simulink model "TorqueControl"  (R2019a)
settings: Solver=FixedStepAuto  StartTime=0.0  StopTime=6  FixedStep=0.015  RelTol=1e-3
undefined symbols (not defined in the file): f_sw, Q_rr, r_c, r_D, u_ce0, u_D0
libraries: Lib_Solve_SSNRSolverJC_TMATS x2, simulink x1
settings Model: Creator=gfretti  LastModifiedBy=gfretti

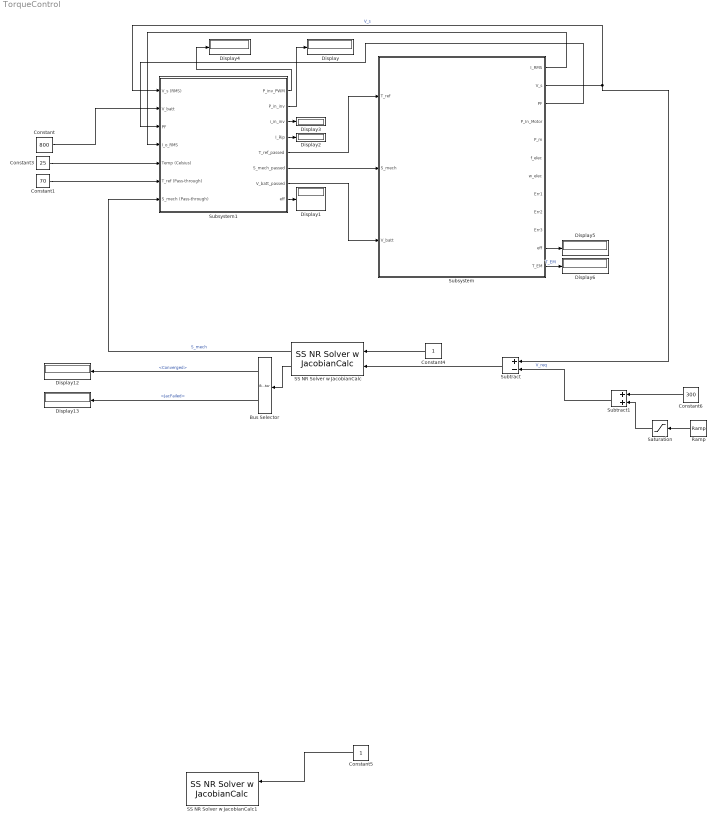
== system TorqueControl ==
  Bus Selector : BusSelector  OutputSignals=Converged,JacFailed
  Constant : Constant  Value=800
  Constant1 : Constant  Value=70
  Constant3 : Constant  Value=25
  Constant4 : Constant
  Constant5 : Constant
  Constant6 : Constant  Value=300
  Display{,1..6,12..13} (9 alike) : Display
  Ramp : simulink/Sources/Ramp  slope=25  start=2  InitialOutput=0
  SS NR Solver w JacobianCalc : Lib_Solve_SSNRSolverJC_TMATS/SS NR Solver w JacobianCalc  SJac_Per_M=[-0.1;-0.01;0.01;0.1]  SNR_IC_M=100  SNR_DX_M=100  SNR_Mx_M=100000  SNR_Mn_M=0.00001  SJacobianAttempts_M=2*10^5  Cond_Limits_M=0.01
  SS NR Solver w JacobianCalc1 : Lib_Solve_SSNRSolverJC_TMATS/SS NR Solver w JacobianCalc  SJac_Per_M=[-0.01;0.01]  SNR_IC_M=150  SNR_DX_M=100  SNR_Mx_M=100000  SNR_Mn_M=0.00001  SJacobianAttempts_M=20000  Cond_Limits_M=0.01
  Saturation : Saturate  UpperLimit=50
  Subsystem : Subsystem  mask{pp=2, flux_m=0.57773, R_s=0.032, L_s=0.00115, P_Fe_Nom=904.3614, S_nom=3000, T_nom=70, P_out_max=22000, I_max=36.5, P_in_max=30000, T_max=80, Poles_i=4, R_s_i=.032, L_s_i=.00086+0.00029, S_nom_i=3000, T_nom_i=70, P_out_max_i=22000, I_max_i=36.5, P_in_max_i=30000, K_i=121, V_nom_i=368, T_max_i=80, CalculatePFe=Compute iron losses automatically, P_Fe_Nom_i=0, I_nom_i=36.5, PF_nom_i=0.99, P_Fe_Calc_Flag=1}
      mask prompts: pp "Pole Pairs"; flux_m "Magnet Flux (wb)"; R_s "Stator Resistance (Ohm)"; L_s "Stator Inductance (H)"; P_Fe_Nom "Iron Losses at Nominal Speed (W)"; S_nom "Nominal Speed (RPM)"; T_nom "Maximum/Nominal reference torque (Nm)"; P_out_max "Maximum output power (W)"; I_max "Currrent Limit"; P_in_max "Input power limit"; T_max "Maximum allowable torque"; Poles_i "Number of poles"; R_s_i "Stator Resistance (Ohm)"; L_s_i "Stator Inductance (H)"; S_nom_i "Nominal Speed (RPM)"; T_nom_i "Maximum/Nominal reference torque (Nm)"; P_out_max_i "Maximum/Nominal output power (W)"; I_max_i "Currrent Limit"; P_in_max_i "Input power limit"; K_i "Back EMF Constant (V/kRPM)"; V_nom_i "Nominal Voltage"; T_max_i "Maximum allowable torque"; P_Fe_Nom_i "Iron Loss at Nominal Conditions"; I_nom_i "Nominal Current"; PF_nom_i "Nominal power factor"
      mask TypeOptions CalculatePFe: Compute iron losses automatically | Input iron losses manually
      mask Callback CalculatePFe:
      | %Create mask parameter objects:
      | PFeMode = get_param(gcb,'CalculatePFe');
      | % P_Fe_Calc_Flag = get_param(gcb,'P_Fe_Calc_Flag');
      | 
      | %Returns cell array of visibility 'on'/'off' strings for all mask
      | %parameters:
      | vis = get_param(gcb,'MaskVisibilities');
      | 
      | if strcmp(PFeMode(1),'I') == 1
      |     %User selects custom ripple option:
      |     visOn = vis;
      |     visOn(24) = {'on'};
      |     visOn(25) = {'off'};
      |     visOn(26) = {'off'};
      |     visOn(27) = {'off'};
      |     %Update mask visibilities:
      |     set_param(gcb,'MaskVisibilities',visOn);
      |     Calculate_Pe_Fe_Flag = 0;
      |     set_param(gcb,'P_Fe_Calc_Flag','0');
      | else
      |     visOff = vis;
      |     visOff(24) = {'off'};
      |     visOff(25) = {'on'};
      |     visOff(26) = {'on'};
      |     visOff(27) = {'off'};
      |     Calculate_Pe_Fe_Flag = 1;
      |     set_param(gcb,'MaskVisibilities',visOff);
      |     set_param(gcb,'P_Fe_Calc_Flag','1');
      | end
      mask DialogControl Container13 Prompt: Tab
      mask DialogControl Container12 Prompt: iDesign
      mask DialogControl Control3 Prompt: Entering zero for resistance or inductance will cause iDesign to use statistical analysis of a set of 400V PMSMs in order to estimate a reasonable resistance and inductance.
      mask DialogControl Container14 Prompt: Iron Loss Calculation
      mask DialogControl run Prompt: RUN IDESIGN
      mask DialogControl run Callback: run('Run_iDesign_SS_PMSM')
  Subsystem1 : Subsystem  mask{T_M=[25 175], u_D_M=[1.16666666666667 0.999999999999999], u_ce0_M=[0.971428571428572 0.848275862068966], R_c_M=[0.0285714285714286 0.0551724137931034], R_D_M=[0.0238095238095238 0.0294117647058824], E0_M=[5.99999999999998e-05 5.99999999999998e-05], E1_M=[5.6e-05 5.6e-05], f_sw_M=20000, L_s_M=0.00115, P_max_I=22000, V_phase_I=400, f_sw_I=0, L_s_I=.00086+0.00029}
      mask prompts: T_M "Temperature Breakpoints (degrees C)"; u_D_M "u_D (Diode voltage at 0A), as a function of T"; u_ce0_M "u_ce0 (IGBT voltage at 0A), as a function of T"; R_c_M "R_c (IGBT resistance), as a function of T"; R_D_M "R_D (Diode resistance), as a linear of T"; E0_M "E0 switching energy coefficient"; E1_M "E1 switching energy coefficient"; f_sw_M "Switching Frequency (Hz)"; L_s_M "Stator Inductance of Attached Motor"; P_max_I "Maximum power"; V_phase_I "Maximum phase voltage (set to 0 to disregard)"; f_sw_I "F_sw (set to 0 to default to maximum for given IGBT)"; L_s_I "Stator inductance of Motor (required for ripple current calculation)"
      mask DialogControl Container4 Prompt: Parameters
      mask DialogControl Control2 Prompt: The way that the above parameters are used is that each vector is 2 long, using points in the linear zone of the curves. Interpolation is used to find values at other temperatures.
      mask DialogControl Container4_copy Prompt: iDesign 1
      mask DialogControl runbutton Prompt: RUN iDESIGN
      mask DialogControl runbutton Callback: run('Run_iDesign_InverterSS')
  Subtract : Sum  Inputs=+-
  Subtract1 : Sum
  wires:
  Subsystem1/5(T_ref_passed) -> Subsystem/1(T_ref)
  Subsystem1/6(S_mech_passed) -> Subsystem/2(S_mech)
  Subsystem1/7(V_batt_passed) -> Subsystem/3(V_batt)
  Subsystem/2(V_s) -> Subtract/1, Subsystem1/1("V_s (RMS) ")  "V_s"
  Subsystem/3(PF) -> Subsystem1/3(PF)
  Constant/1 -> Subsystem1/2(V_batt)
  Subsystem1/2(P_in_inv) -> Display/1
  Subsystem1/8(eff) -> Display1/1
  Subsystem1/4(I_Rip) -> Display2/1
  Subsystem1/3(i_in_inv) -> Display3/1
  Subsystem1/1(P_inv_PWM) -> Display4/1
  Subsystem/11(eff) -> Display5/1
  Constant3/1 -> Subsystem1/5(Temp (Celsius))
  Subsystem/1("I_RMS ") -> Subsystem1/4(I_o_RMS)
  Bus Selector/1 -> Display12/1  "<Converged>"
  Bus Selector/2 -> Display13/1  "<JacFailed>"
  SS NR Solver w JacobianCalc/2 -> Bus Selector/1
  Constant5/1 -> SS NR Solver w JacobianCalc1/1
  ? -> SS NR Solver w JacobianCalc1/2
  Constant4/1 -> SS NR Solver w JacobianCalc/1
  Subtract/1 -> SS NR Solver w JacobianCalc/2
  Constant1/1 -> Subsystem1/6(T_ref (Pass-through))
  SS NR Solver w JacobianCalc/1 -> Subsystem1/7(S_mech (Pass-through))  "S_mech"
  Subsystem/12(T_EM) -> Display6/1  "T_EM"
  Subtract1/1 -> Subtract/2  "V_req"
  Constant6/1 -> Subtract1/1
  Ramp/1 -> Saturation/1
  Saturation/1 -> Subtract1/2

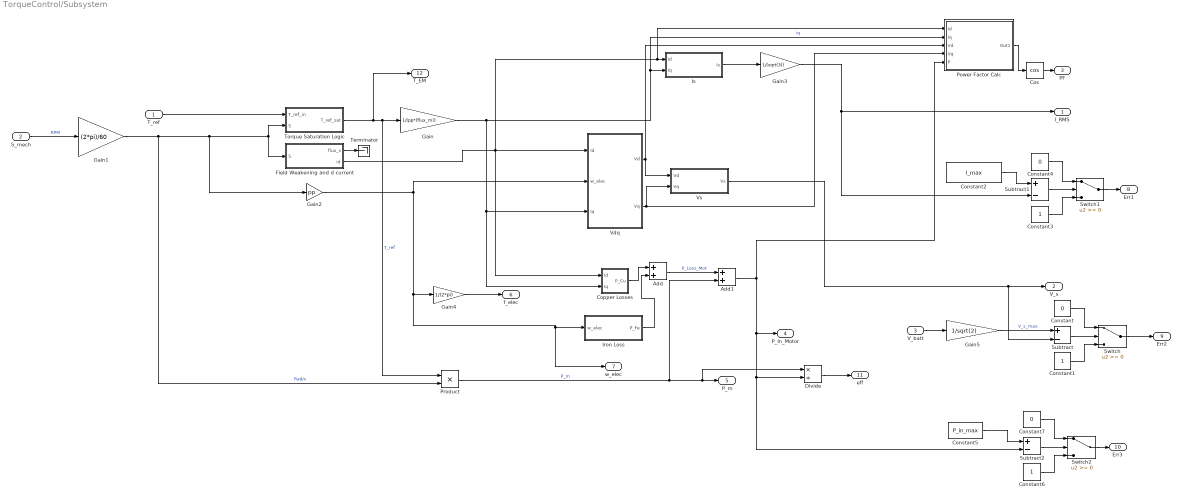
== system TorqueControl/Subsystem ==
  T_ref : Inport
  S_mech : Inport  Port=2
  V_batt : Inport  Port=3
  Add : Sum
  Add1 : Sum
  Constant : Constant  Value=0
  Constant1 : Constant
  Constant2 : Constant  Value=I_max
  Constant3 : Constant
  Constant4 : Constant  Value=0
  Constant5 : Constant  Value=P_in_max
  Constant6 : Constant
  Constant7 : Constant  Value=0
  Copper Losses : Subsystem
  Cos : Trigonometry  Operator=cos
  Divide : Product  Inputs=*/
  "Field Weakening and d current " : Subsystem
  Gain : Gain  Gain=1/(pp*(flux_m))
  Gain1 : Gain  Gain=(2*pi)/60
  Gain2 : Gain  Gain=pp
  Gain3 : Gain  Gain=1/(sqrt(3))
  Gain4 : Gain  Gain=1/(2*pi)
  Gain5 : Gain  Gain=1/sqrt(2)
  Iron Loss : Subsystem
  Is : Subsystem
  "Power Factor Calc " : Subsystem
  Product : Product
  Subtract : Sum  Inputs=+-
  Subtract1 : Sum  Inputs=+-
  Subtract2 : Sum  Inputs=+-
  Switch : Switch
  Switch1 : Switch
  Switch2 : Switch
  Terminator : Terminator
  Torque Saturation Logic : Subsystem
  Vdq : Subsystem
  Vs : Subsystem
  "I_RMS " : Outport
  V_s : Outport  Port=2
  PF : Outport  Port=3
  P_In_Motor : Outport  Port=4
  P_m : Outport  Port=5
  f_elec : Outport  Port=6
  w_elec : Outport  Port=7
  Err1 : Outport  Port=8
  Err2 : Outport  Port=9
  Err3 : Outport  Port=10
  eff : Outport  Port=11
  T_EM : Outport  Port=12
  wires:
  S_mech/1 -> Gain1/1  "RPM"
  T_ref/1 -> Torque Saturation Logic/1(T_ref_in)
  "Field Weakening and d current "/2(id) -> Copper Losses/1(Id), "Power Factor Calc "/1(Id), Is/1(Id), Vdq/1(Id)
  Gain3/1 -> Subtract1/2, "I_RMS "/1
  Gain2/1 -> Vdq/2(w_elec), Gain4/1, w_elec/1, Iron Loss/1(w_elec)
  Torque Saturation Logic/1(T_ref_sat) -> T_EM/1, Product/1, Gain/1  "T_ref"
  Gain/1 -> "Power Factor Calc "/2(Iq), Is/2(Iq), Copper Losses/2(Iq), Vdq/3(Iq)  "iq"
  Gain1/1 -> Product/2, Gain2/1, "Field Weakening and d current "/1(S), Torque Saturation Logic/2(S)  "Rad/s"
  Copper Losses/1(P_Cu) -> Add/1
  Iron Loss/1(P_Fe) -> Add/2
  Add/1 -> Add1/1  "P_Loss_Mot"
  Product/1 -> Add1/2, Divide/1, P_m/1  "P_m"
  Vdq/1(Vd) -> Vs/1(Vd), "Power Factor Calc "/3(Vd)
  Vdq/2(Vq) -> "Power Factor Calc "/4(Vq), Vs/2(Vq)
  Is/1(Is) -> Gain3/1
  Vs/1(Vs) -> Subtract/2, V_s/1
  "Power Factor Calc "/1(Out1) -> Cos/1
  Add1/1 -> Divide/2, Subtract2/2, P_In_Motor/1, "Power Factor Calc "/5(P)
  Gain4/1 -> f_elec/1
  V_batt/1 -> Gain5/1
  Gain5/1 -> Subtract/1  "V_s_max"
  Subtract/1 -> Switch/2
  Constant/1 -> Switch/1
  Constant1/1 -> Switch/3
  Switch/1 -> Err2/1
  Constant2/1 -> Subtract1/1
  Switch1/1 -> Err1/1
  Constant3/1 -> Switch1/3
  Constant4/1 -> Switch1/1
  Subtract1/1 -> Switch1/2
  Switch2/1 -> Err3/1
  Constant7/1 -> Switch2/1
  Constant5/1 -> Subtract2/1
  Subtract2/1 -> Switch2/2
  Constant6/1 -> Switch2/3
  Divide/1 -> eff/1
  Cos/1 -> PF/1
  "Field Weakening and d current "/1(flux_s) -> Terminator/1

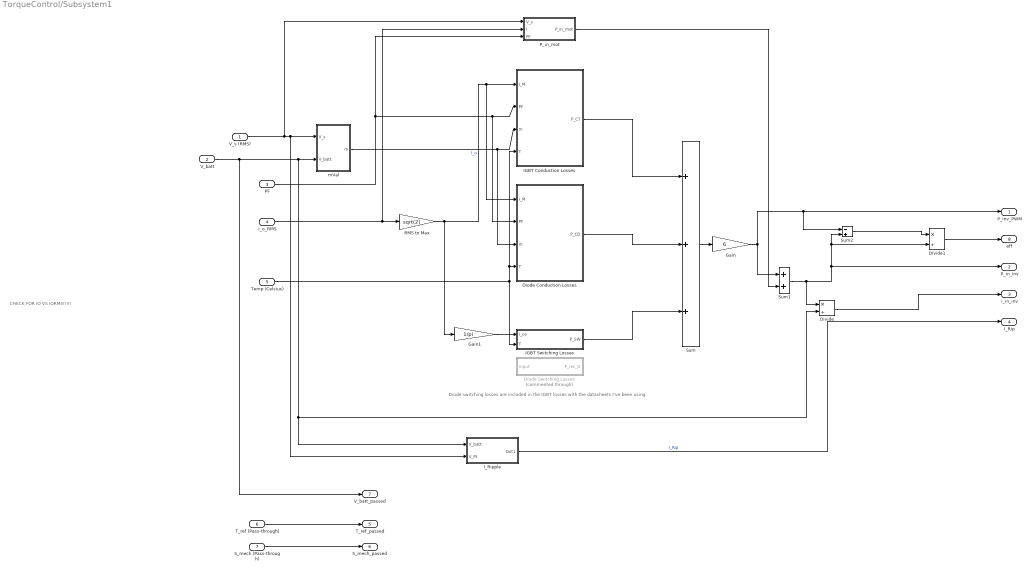
== system TorqueControl/Subsystem1 ==
  note: Diode switching losses are included in the IGBT losses with the datasheets I've been using
  note: CHECK FOR IO VS IORMS!!!!!
  "V_s (RMS) " : Inport
  V_batt : Inport  Port=2
  PF : Inport  Port=3
  I_o_RMS : Inport  Port=4
  Temp (Celsius) : Inport  Port=5
  T_ref (Pass-through) : Inport  Port=6
  S_mech (Pass-through) : Inport  Port=7
  Diode Conduction Losses : Subsystem
  Diode Switching Losses : Subsystem  Commented=through
  Divide : Product  Inputs=*/
  Divide1 : Product  Inputs=*/
  Gain : Gain  Gain=6
  Gain1 : Gain  Gain=1/pi
  IGBT Conduction Losses : Subsystem
  IGBT Switching Losses : Subsystem
  I_Ripple : Subsystem
  P_in_mot : Subsystem
  RMS to Max : Gain  Gain=sqrt(2)
  Sum : Sum  Inputs=+++
  Sum1 : Sum
  Sum2 : Sum  Inputs=-+
  mVal : Subsystem
  P_inv_PWM : Outport
  P_in_inv : Outport  Port=2
  i_in_inv : Outport  Port=3
  I_Rip : Outport  Port=4
  T_ref_passed : Outport  Port=5
  S_mech_passed : Outport  Port=6
  V_batt_passed : Outport  Port=7
  eff : Outport  Port=8
  wires:
  I_o_RMS/1 -> P_in_mot/2(I), RMS to Max/1
  RMS to Max/1 -> Gain1/1, Diode Conduction Losses/1(I_M), IGBT Conduction Losses/1(I_M)  "I_o"
  V_batt/1 -> V_batt_passed/1, mVal/2(V_batt), I_Ripple/1(V_batt), Divide/2
  IGBT Conduction Losses/1(P_CT) -> Sum/1
  Sum/1 -> Gain/1
  Gain/1 -> Sum2/1, P_inv_PWM/1, Sum1/1
  PF/1 -> P_in_mot/3(PF), Diode Conduction Losses/2(PF), IGBT Conduction Losses/2(PF)
  mVal/1(m) -> Diode Conduction Losses/3(m), IGBT Conduction Losses/3(m)
  "V_s (RMS) "/1 -> P_in_mot/1(V_s), I_Ripple/2("V_M "), mVal/1(V_s)
  P_in_mot/1(P_in_mot) -> Sum1/2
  Divide/1 -> i_in_inv/1
  Gain1/1 -> IGBT Switching Losses/1(I_ce)
  IGBT Switching Losses/1(P_SW) -> Sum/3
  Diode Conduction Losses/1(P_CD) -> Sum/2
  Temp (Celsius)/1 -> IGBT Switching Losses/2(T), Diode Conduction Losses/4(T), IGBT Conduction Losses/4(T)
  I_Ripple/1(Out1) -> I_Rip/1  "I_Rip"
  T_ref (Pass-through)/1 -> T_ref_passed/1
  S_mech (Pass-through)/1 -> S_mech_passed/1
  Sum1/1 -> Divide/1, Sum2/2, Divide1/2, P_in_inv/1
  Sum2/1 -> Divide1/1
  Divide1/1 -> eff/1

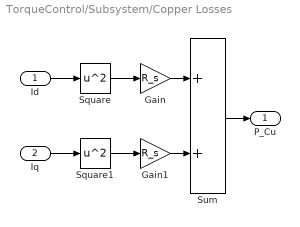
== system TorqueControl/Subsystem/Copper Losses ==
  Id : Inport
  Iq : Inport  Port=2
  Gain : Gain  Gain=R_s
  Gain1 : Gain  Gain=R_s
  Square : Math  Operator=square  SaturateOnIntegerOverflow=on
  Square1 : Math  Operator=square  SaturateOnIntegerOverflow=on
  Sum : Sum
  P_Cu : Outport
  wires:
  Iq/1 -> Square1/1
  Id/1 -> Square/1
  Square/1 -> Gain/1
  Square1/1 -> Gain1/1
  Gain1/1 -> Sum/2
  Gain/1 -> Sum/1
  Sum/1 -> P_Cu/1

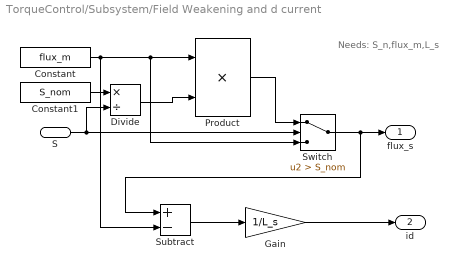
== system TorqueControl/Subsystem/Field Weakening and d current  ==
  note: Needs: S_n,flux_m,L_s
  S : Inport
  Constant : Constant  Value=flux_m
  Constant1 : Constant  Value=S_nom
  Divide : Product  Inputs=*/
  Gain : Gain  Gain=1/L_s
  Product : Product
  Subtract : Sum  Inputs=+-
  Switch : Switch  Criteria=u2 > Threshold  Threshold=S_nom
  flux_s : Outport
  id : Outport  Port=2
  wires:
  S/1 -> Divide/2, Switch/2
  Product/1 -> Switch/1
  Constant1/1 -> Divide/1
  Divide/1 -> Product/2
  Constant/1 -> Switch/3, Product/1, Subtract/2
  Switch/1 -> Subtract/1, flux_s/1
  Subtract/1 -> Gain/1
  Gain/1 -> id/1

== system TorqueControl/Subsystem/Iron Loss ==
  w_elec : Inport
  Constant : Constant  Value=S_nom*((2*pi)/60)*pp
  Divide : Product  Inputs=*/
  Gain : Gain  Gain=P_Fe_Nom
  P_Fe : Outport
  wires:
  Gain/1 -> P_Fe/1
  w_elec/1 -> Divide/1
  Constant/1 -> Divide/2
  Divide/1 -> Gain/1

== system TorqueControl/Subsystem/Is ==
  Id : Inport
  Iq : Inport  Port=2
  Add : Sum
  Square : Math  Operator=square  SaturateOnIntegerOverflow=on
  Square Root : Sqrt  SaturateOnIntegerOverflow=on
  Square1 : Math  Operator=square  SaturateOnIntegerOverflow=on
  Is : Outport
  wires:
  Iq/1 -> Square/1
  Id/1 -> Square1/1
  Square1/1 -> Add/1
  Square/1 -> Add/2
  Add/1 -> Square Root/1
  Square Root/1 -> Is/1

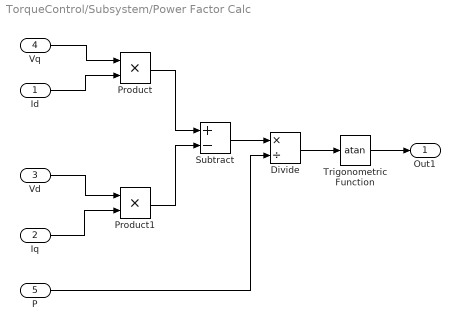
== system TorqueControl/Subsystem/Power Factor Calc  ==
  Id : Inport
  Iq : Inport  Port=2
  Vd : Inport  Port=3
  Vq : Inport  Port=4
  P : Inport  Port=5
  Divide : Product  Inputs=*/
  Product : Product
  Product1 : Product
  Subtract : Sum  Inputs=+-
  Trigonometric Function : Trigonometry  Operator=atan
  Out1 : Outport
  wires:
  Vq/1 -> Product/1
  Id/1 -> Product/2
  Vd/1 -> Product1/1
  Iq/1 -> Product1/2
  Product1/1 -> Subtract/2
  Product/1 -> Subtract/1
  Subtract/1 -> Divide/1
  P/1 -> Divide/2
  Divide/1 -> Trigonometric Function/1
  Trigonometric Function/1 -> Out1/1

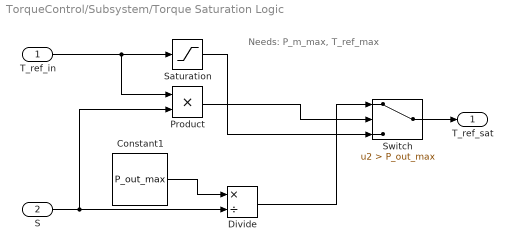
== system TorqueControl/Subsystem/Torque Saturation Logic ==
  note: Needs: P_m_max, T_ref_max
  T_ref_in : Inport
  S : Inport  Port=2
  Constant1 : Constant  Value=P_out_max
  Divide : Product  Inputs=*/
  Product : Product
  Saturation : Saturate  UpperLimit=T_nom  LowerLimit=0
  Switch : Switch  Criteria=u2 > Threshold  Threshold=P_out_max
  T_ref_sat : Outport
  wires:
  T_ref_in/1 -> Product/1, Saturation/1
  Constant1/1 -> Divide/1
  S/1 -> Product/2, Divide/2
  Saturation/1 -> Switch/3
  Product/1 -> Switch/2
  Divide/1 -> Switch/1
  Switch/1 -> T_ref_sat/1

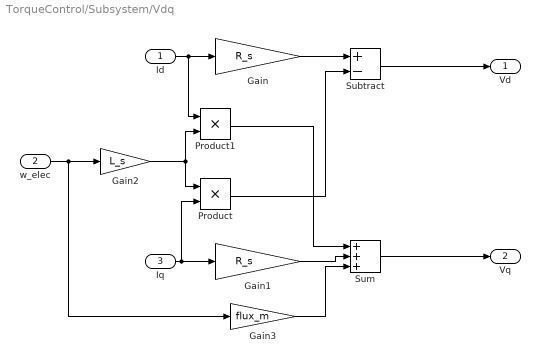
== system TorqueControl/Subsystem/Vdq ==
  Id : Inport
  w_elec : Inport  Port=2
  Iq : Inport  Port=3
  Gain : Gain  Gain=R_s
  Gain1 : Gain  Gain=R_s
  Gain2 : Gain  Gain=L_s
  Gain3 : Gain  Gain=flux_m
  Product : Product
  Product1 : Product
  Subtract : Sum  Inputs=+-
  Sum : Sum  Inputs=+++
  Vd : Outport
  Vq : Outport  Port=2
  wires:
  Id/1 -> Product1/1, Gain/1
  Iq/1 -> Gain1/1, Product/2
  w_elec/1 -> Gain3/1, Gain2/1
  Gain/1 -> Subtract/1
  Gain2/1 -> Product/1, Product1/2
  Product/1 -> Subtract/2
  Subtract/1 -> Vd/1
  Product1/1 -> Sum/1
  Gain1/1 -> Sum/2
  Gain3/1 -> Sum/3
  Sum/1 -> Vq/1

== system TorqueControl/Subsystem/Vs ==
  Vd : Inport
  Vq : Inport  Port=2
  Add : Sum
  Square : Math  Operator=square  SaturateOnIntegerOverflow=on
  Square Root : Sqrt  SaturateOnIntegerOverflow=on
  Square1 : Math  Operator=square  SaturateOnIntegerOverflow=on
  Vs : Outport
  wires:
  Vq/1 -> Square/1
  Vd/1 -> Square1/1
  Square1/1 -> Add/1
  Square/1 -> Add/2
  Add/1 -> Square Root/1
  Square Root/1 -> Vs/1

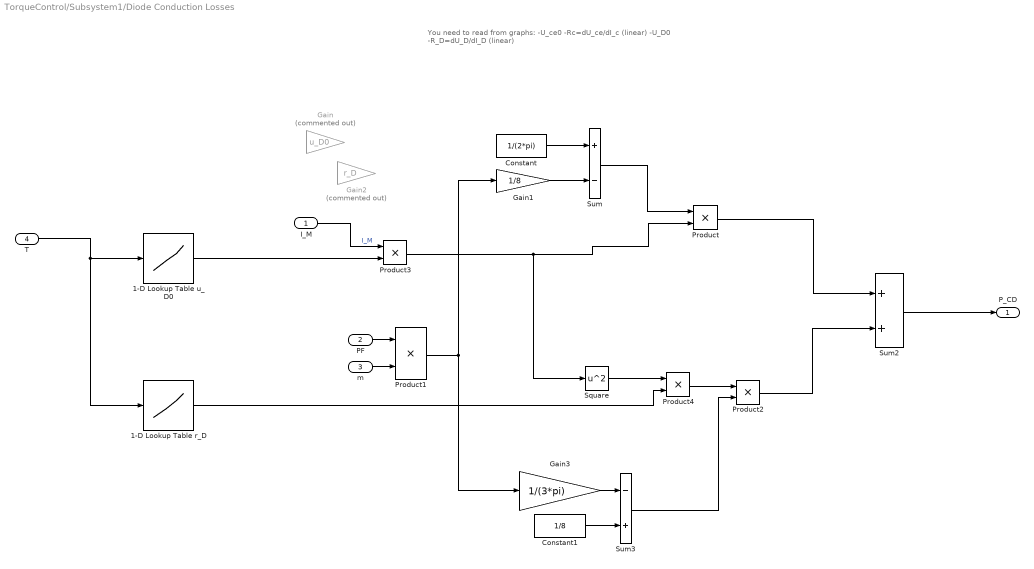
== system TorqueControl/Subsystem1/Diode Conduction Losses ==
  note: You need to read from graphs:
      |
      | -U_ce0
      | -Rc=dU_ce/dI_c (linear)
      | -U_D0
      | -R_D=dU_D/dI_D (linear)
  I_M : Inport
  PF : Inport  Port=2
  m : Inport  Port=3
  T : Inport  Port=4
  1-D Lookup Table r_D : Lookup_n-D  NumberOfTableDimensions=1  BreakpointsForDimension1=T_M  Table=R_D_M  InternalRulePriority=Speed  RndMeth=Simplest  InputSameDT=on
  1-D Lookup Table u_D0 : Lookup_n-D  NumberOfTableDimensions=1  BreakpointsForDimension1=T_M  Table=u_D_M  InternalRulePriority=Speed  RndMeth=Simplest  InputSameDT=on
  Constant : Constant  Value=1/(2*pi)
  Constant1 : Constant  Value=1/8
  Gain : Gain  Commented=on  Gain=u_D0
  Gain1 : Gain  Gain=1/8
  Gain2 : Gain  Commented=on  Gain=r_D
  Gain3 : Gain  Gain=1/(3*pi)
  Product{,1..4} (5 alike) : Product
  Square : Math  Operator=square  SaturateOnIntegerOverflow=on
  Sum : Sum  Inputs=+-
  Sum2 : Sum
  Sum3 : Sum  Inputs=-+
  P_CD : Outport
  wires:
  Product/1 -> Sum2/1
  Product2/1 -> Sum2/2
  Sum2/1 -> P_CD/1
  I_M/1 -> Product3/1  "I_M"
  Product3/1 -> Product/2, Square/1
  Constant/1 -> Sum/1
  PF/1 -> Product1/1
  m/1 -> Product1/2
  Gain1/1 -> Sum/2
  Product1/1 -> Gain3/1, Gain1/1
  Sum/1 -> Product/1
  Square/1 -> Product4/1
  Gain3/1 -> Sum3/1
  Product4/1 -> Product2/1
  Constant1/1 -> Sum3/2
  Sum3/1 -> Product2/2
  T/1 -> 1-D Lookup Table u_D0/1, 1-D Lookup Table r_D/1
  1-D Lookup Table u_D0/1 -> Product3/2
  1-D Lookup Table r_D/1 -> Product4/2

== system TorqueControl/Subsystem1/Diode Switching Losses ==
  note: I_Drrpeak=2Qrr/trr
  note: Worst case - voltage across diode is supply voltage
  Input : Inport
  Constant1 : Constant  Value=f_sw
  Gain : Gain  Gain=.25*Q_rr
  Product2 : Product
  P_rec_D : Outport
  wires:
  Product2/1 -> P_rec_D/1
  Constant1/1 -> Product2/2  "I_M"
  Gain/1 -> Product2/1
  Input/1 -> Gain/1  "V_batt"

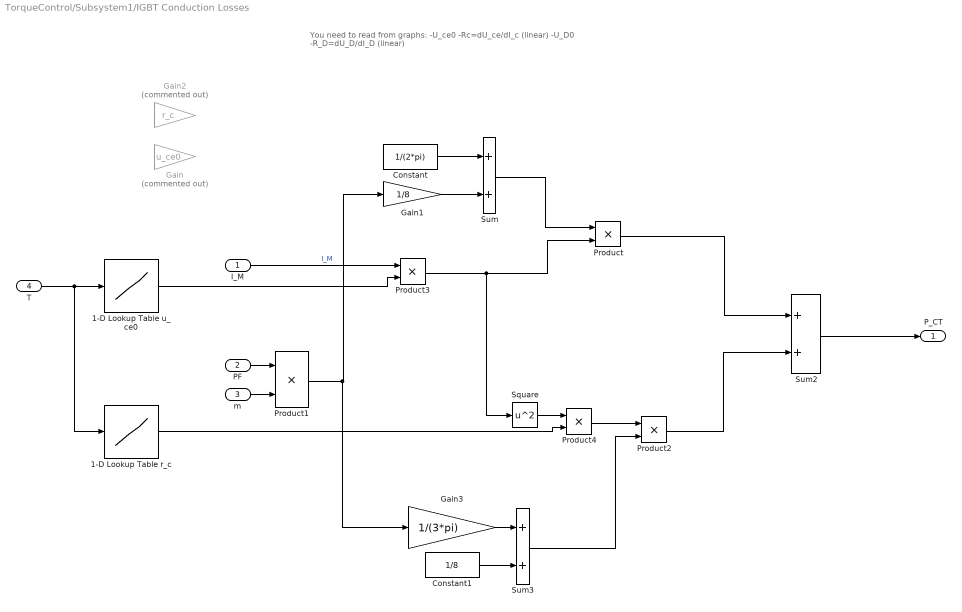
== system TorqueControl/Subsystem1/IGBT Conduction Losses ==
  note: You need to read from graphs:
      |
      | -U_ce0
      | -Rc=dU_ce/dI_c (linear)
      | -U_D0
      | -R_D=dU_D/dI_D (linear)
  I_M : Inport
  PF : Inport  Port=2
  m : Inport  Port=3
  T : Inport  Port=4
  1-D Lookup Table r_c : Lookup_n-D  NumberOfTableDimensions=1  BreakpointsForDimension1=T_M  Table=R_c_M  InternalRulePriority=Speed  RndMeth=Simplest  InputSameDT=on
  1-D Lookup Table u_ce0 : Lookup_n-D  NumberOfTableDimensions=1  BreakpointsForDimension1=T_M  Table=u_ce0_M  InternalRulePriority=Speed  RndMeth=Simplest  InputSameDT=on
  Constant : Constant  Value=1/(2*pi)
  Constant1 : Constant  Value=1/8
  Gain : Gain  Commented=on  Gain=u_ce0
  Gain1 : Gain  Gain=1/8
  Gain2 : Gain  Commented=on  Gain=r_c
  Gain3 : Gain  Gain=1/(3*pi)
  Product{,1..4} (5 alike) : Product
  Square : Math  Operator=square  SaturateOnIntegerOverflow=on
  Sum : Sum
  Sum2 : Sum
  Sum3 : Sum
  P_CT : Outport
  wires:
  Product/1 -> Sum2/1
  Product2/1 -> Sum2/2
  Sum2/1 -> P_CT/1
  I_M/1 -> Product3/1  "I_M"
  Product3/1 -> Product/2, Square/1
  Constant/1 -> Sum/1
  PF/1 -> Product1/1
  m/1 -> Product1/2
  Gain1/1 -> Sum/2
  Product1/1 -> Gain3/1, Gain1/1
  Sum/1 -> Product/1
  Square/1 -> Product4/1
  Gain3/1 -> Sum3/1
  Product4/1 -> Product2/1
  Constant1/1 -> Sum3/2
  Sum3/1 -> Product2/2
  T/1 -> 1-D Lookup Table u_ce0/1, 1-D Lookup Table r_c/1
  1-D Lookup Table u_ce0/1 -> Product3/2
  1-D Lookup Table r_c/1 -> Product4/2

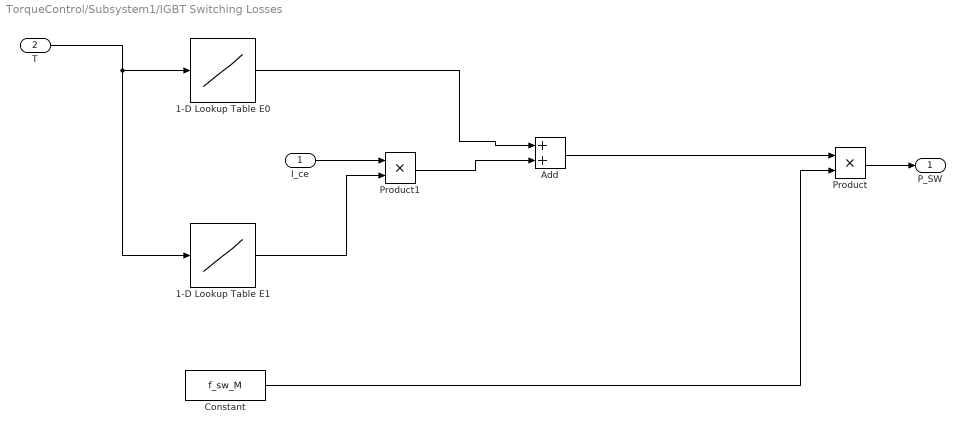
== system TorqueControl/Subsystem1/IGBT Switching Losses ==
  I_ce : Inport
  T : Inport  Port=2
  1-D Lookup Table E0 : Lookup_n-D  NumberOfTableDimensions=1  BreakpointsForDimension1=T_M  Table=E0_M  InternalRulePriority=Speed  RndMeth=Simplest  InputSameDT=on
  1-D Lookup Table E1 : Lookup_n-D  NumberOfTableDimensions=1  BreakpointsForDimension1=T_M  Table=E1_M  InternalRulePriority=Speed  RndMeth=Simplest  InputSameDT=on
  Add : Sum
  Constant : Constant  Value=f_sw_M
  Product : Product
  Product1 : Product
  P_SW : Outport
  wires:
  Constant/1 -> Product/2
  Product/1 -> P_SW/1
  Add/1 -> Product/1
  I_ce/1 -> Product1/1
  1-D Lookup Table E0/1 -> Add/1
  Product1/1 -> Add/2
  T/1 -> 1-D Lookup Table E0/1, 1-D Lookup Table E1/1
  1-D Lookup Table E1/1 -> Product1/2

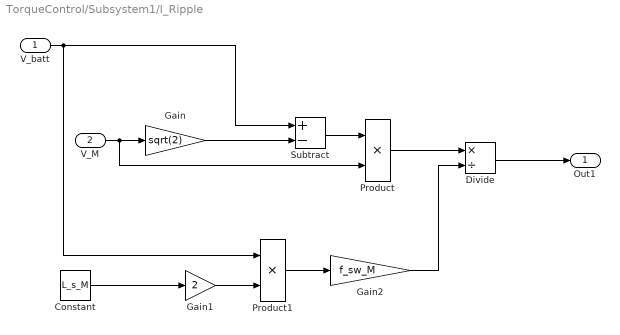
== system TorqueControl/Subsystem1/I_Ripple ==
  V_batt : Inport
  "V_M " : Inport  Port=2
  Constant : Constant  Value=L_s_M
  Divide : Product  Inputs=*/
  Gain : Gain  Gain=sqrt(2)
  Gain1 : Gain  Gain=2
  Gain2 : Gain  Gain=f_sw_M
  Product : Product
  Product1 : Product
  Subtract : Sum  Inputs=+-
  Out1 : Outport
  wires:
  "V_M "/1 -> Product/2, Gain/1
  Gain/1 -> Subtract/2
  V_batt/1 -> Subtract/1, Product1/1
  Subtract/1 -> Product/1
  Product/1 -> Divide/1
  Constant/1 -> Gain1/1
  Gain1/1 -> Product1/2
  Product1/1 -> Gain2/1
  Gain2/1 -> Divide/2
  Divide/1 -> Out1/1

== system TorqueControl/Subsystem1/P_in_mot ==
  V_s : Inport
  I : Inport  Port=2
  PF : Inport  Port=3
  Gain : Gain  Gain=sqrt(3)
  Product : Product  Inputs=3
  P_in_mot : Outport
  wires:
  I/1 -> Product/2
  PF/1 -> Product/3
  V_s/1 -> Product/1
  Gain/1 -> P_in_mot/1
  Product/1 -> Gain/1

== system TorqueControl/Subsystem1/mVal ==
  V_s : Inport
  V_batt : Inport  Port=2
  Divide : Product  Inputs=*/
  Gain : Gain  Gain=sqrt(2)
  m : Outport
  wires:
  Divide/1 -> m/1
  V_s/1 -> Gain/1
  Gain/1 -> Divide/1
  V_batt/1 -> Divide/2
